simulink model "regler_pedal_img"  (R2012b)
settings: Solver=ode45  StartTime=0.0  StopTime=10.0  RelTol=1e-3
values from neighbouring files (symbols this model uses):
  n_r = 2    [Init_Project1.m]    (also in Init_Project2.m)
  V_D = 2.290 *10^-3    (= 0.00229)    [Init_Project1.m]    (also in Init_Project2.m = n_cyl*V_d)
undefined symbols (not defined in the file or in its folder): C_p, TqEvsNe
settings Model: Creator=rasme879  LastModifiedBy=rasme879

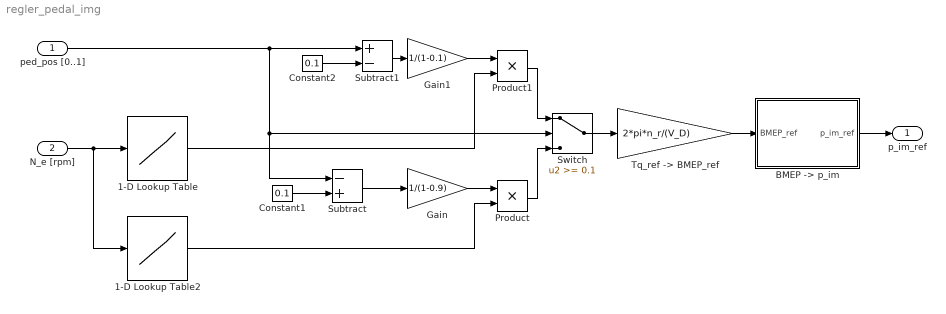
== system regler_pedal_img ==
  ped_pos [0..1] : Inport
  N_e [rpm] : Inport  Port=2
  1-D Lookup Table : Lookup_n-D  NumberOfTableDimensions=1  BreakpointsForDimension1=TqEvsNe.Ne  Table=TqEvsNe.TqMAX  RndMeth=Simplest  InputSameDT=on
  1-D Lookup Table2 : Lookup_n-D  NumberOfTableDimensions=1  BreakpointsForDimension1=TqEvsNe.Ne  Table=TqEvsNe.TqMIN  RndMeth=Simplest  InputSameDT=on
  "BMEP -> p_im" : Subsystem
  Constant1 : Constant  Value=0.1
  Constant2 : Constant  Value=0.1
  Gain : Gain  Gain=1/(1-0.9)
  Gain1 : Gain  Gain=1/(1-0.1)
  Product : Product  RndMeth=Zero
  Product1 : Product  RndMeth=Zero
  Subtract : Sum  Inputs=-+
  Subtract1 : Sum  Inputs=+-
  Switch : Switch  Threshold=0.1
  "Tq_ref -> BMEP_ref" : Gain  Gain=2*pi*n_r/(V_D)
  p_im_ref : Outport
  wires:
  ped_pos [0..1]/1 -> Subtract/1, Switch/2, Subtract1/1
  N_e [rpm]/1 -> 1-D Lookup Table2/1, 1-D Lookup Table/1
  Constant1/1 -> Subtract/2
  Subtract/1 -> Gain/1
  Gain/1 -> Product/1
  Constant2/1 -> Subtract1/2
  Subtract1/1 -> Gain1/1
  Gain1/1 -> Product1/1
  1-D Lookup Table/1 -> Product1/2
  1-D Lookup Table2/1 -> Product/2
  Product1/1 -> Switch/1
  Product/1 -> Switch/3
  Switch/1 -> "Tq_ref -> BMEP_ref"/1
  "Tq_ref -> BMEP_ref"/1 -> "BMEP -> p_im"/1(BMEP_ref)
  "BMEP -> p_im"/1(p_im_ref) -> p_im_ref/1

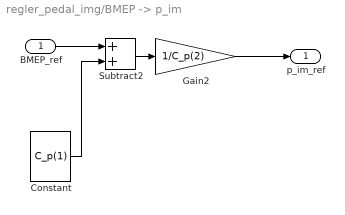
== system regler_pedal_img/BMEP -> p_im ==
  BMEP_ref : Inport
  Constant : Constant  Value=C_p(1)
  Gain2 : Gain  Gain=1/C_p(2)
  Subtract2 : Sum
  p_im_ref : Outport
  wires:
  Subtract2/1 -> Gain2/1
  Gain2/1 -> p_im_ref/1
  BMEP_ref/1 -> Subtract2/1
  Constant/1 -> Subtract2/2
